simulink model "ComplexLS"  (R2018b)
settings: Solver=FixedStepAuto  StartTime=1  StopTime=10  FixedStep=1  RelTol=1e-3
libraries: hdlsllib x11, simulink x1
settings Model: Creator=jason  LastModifiedBy=jason
settings OptimizationCC: DefaultParameterBehavior=Inlined

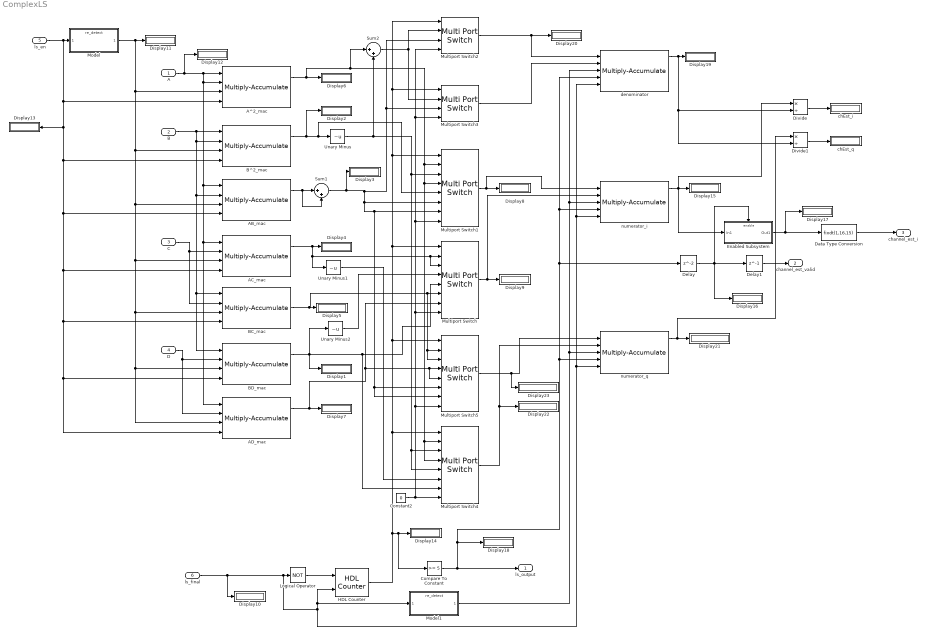
== system ComplexLS ==
  A : Inport  OutDataTypeStr=fixdt(1,16,15)  SampleTime=1  Interpolate=off
  B : Inport  Port=2  OutDataTypeStr=fixdt(1,16,15)  SampleTime=1  Interpolate=off
  C : Inport  Port=3  OutDataTypeStr=fixdt(1,16,15)  SampleTime=1  Interpolate=off
  D : Inport  Port=4  OutDataTypeStr=fixdt(1,16,15)  SampleTime=1  Interpolate=off
  ls_en : Inport  Port=5  OutDataTypeStr=boolean
  ls_final : Inport  Port=6  OutDataTypeStr=boolean
  AB_mac : hdlsllib/HDL Operations/Multiply-Accumulate  opMode=Streaming - using Start and End ports  initValueSetting=Dialog  initValue=0  initValueSetting2=Dialog  initValue2=0  initValueSetting3=Dialog  initValue3=0  num_samples=2  RndMeth2=Floor  RndMeth3=Floor  datatype2=fixdt(1,64,32)  datatype3=Inherit: Inherit via back propagation  validOut=on  endInandOut=off  startOut=off  countOut=on  dim=-1  DoSatur=off  parallel=off
      settings: SourceProductName=HDL Coder  SourceProductBaseCode=HD
  AC_mac : hdlsllib/HDL Operations/Multiply-Accumulate  opMode=Streaming - using Start and End ports  initValueSetting=Dialog  initValue=0  initValueSetting2=Dialog  initValue2=0  initValueSetting3=Dialog  initValue3=0  num_samples=2  RndMeth2=Floor  RndMeth3=Floor  datatype2=fixdt(1,64,32)  datatype3=Inherit: Inherit via back propagation  validOut=on  endInandOut=off  startOut=off  countOut=on  dim=-1  DoSatur=off  parallel=off
      settings: SourceProductName=HDL Coder  SourceProductBaseCode=HD
  AD_mac : hdlsllib/HDL Operations/Multiply-Accumulate  opMode=Streaming - using Start and End ports  initValueSetting=Dialog  initValue=0  initValueSetting2=Dialog  initValue2=0  initValueSetting3=Dialog  initValue3=0  num_samples=2  RndMeth2=Floor  RndMeth3=Floor  datatype2=fixdt(1,64,32)  datatype3=Inherit: Inherit via back propagation  validOut=on  endInandOut=off  startOut=off  countOut=on  dim=-1  DoSatur=off  parallel=off
      settings: SourceProductName=HDL Coder  SourceProductBaseCode=HD
  A^2_mac : hdlsllib/HDL Operations/Multiply-Accumulate  opMode=Streaming - using Start and End ports  initValueSetting=Dialog  initValue=0  initValueSetting2=Dialog  initValue2=0  initValueSetting3=Dialog  initValue3=0  num_samples=2  RndMeth2=Floor  RndMeth3=Floor  datatype2=fixdt(1,64,32)  datatype3=Inherit: Inherit via back propagation  validOut=on  endInandOut=off  startOut=off  countOut=on  dim=-1  DoSatur=off  parallel=off
      settings: SourceProductName=HDL Coder  SourceProductBaseCode=HD
  BC_mac : hdlsllib/HDL Operations/Multiply-Accumulate  opMode=Streaming - using Start and End ports  initValueSetting=Dialog  initValue=0  initValueSetting2=Dialog  initValue2=0  initValueSetting3=Dialog  initValue3=0  num_samples=2  RndMeth2=Floor  RndMeth3=Floor  datatype2=fixdt(1,64,32)  datatype3=Inherit: Inherit via back propagation  validOut=off  endInandOut=off  startOut=off  countOut=on  dim=-1  DoSatur=off  parallel=off
      settings: SourceProductName=HDL Coder  SourceProductBaseCode=HD
  BD_mac : hdlsllib/HDL Operations/Multiply-Accumulate  opMode=Streaming - using Start and End ports  initValueSetting=Dialog  initValue=0  initValueSetting2=Dialog  initValue2=0  initValueSetting3=Dialog  initValue3=0  num_samples=2  RndMeth2=Floor  RndMeth3=Floor  datatype2=fixdt(1,64,32)  datatype3=Inherit: Inherit via back propagation  validOut=on  endInandOut=off  startOut=off  countOut=on  dim=-1  DoSatur=off  parallel=off
      settings: SourceProductName=HDL Coder  SourceProductBaseCode=HD
  B^2_mac : hdlsllib/HDL Operations/Multiply-Accumulate  opMode=Streaming - using Start and End ports  initValueSetting=Dialog  initValue=0  initValueSetting2=Dialog  initValue2=0  initValueSetting3=Dialog  initValue3=0  num_samples=2  RndMeth2=Floor  RndMeth3=Floor  datatype2=fixdt(1,64,32)  datatype3=Inherit: Inherit via back propagation  validOut=on  endInandOut=off  startOut=off  countOut=on  dim=-1  DoSatur=off  parallel=off
      settings: SourceProductName=HDL Coder  SourceProductBaseCode=HD
  Compare To Constant : simulink/Logic and Bit Operations/Compare To Constant  relop=>=  const=5  OutDataTypeStr=boolean
  Constant2 : Constant  Value=0  OutDataTypeStr=fixdt(1,64,32)  SampleTime=-1
  Data Type Conversion : DataTypeConversion  OutDataTypeStr=fixdt(1,16,15)
  Delay : Delay
  Delay1 : Delay  DelayLength=1
  Display{1..23} (23 alike) : Display
  Divide : Product  Inputs=*/  OutDataTypeStr=double  SaturateOnIntegerOverflow=on  RndMeth=Zero
  Divide1 : Product  Inputs=*/  OutDataTypeStr=double  SaturateOnIntegerOverflow=on  RndMeth=Zero
  Enabled Subsystem : Subsystem  TreatAsAtomicUnit=on
  HDL Counter : hdlsllib/Sources/HDL Counter  CountType=Count limited  CountInit=0  CountStep=1  CountMax=5  CountFromType=Initial value  CountFrom=0  CountResetPort=on  CountLoadPort=off  CountEnbPort=on  CountDirPort=off  CountDataType=Unsigned  CountWordLen=8  CountFracLen=0  CountSampTime=1
      settings: SourceProductBaseCode=HD
  Logical Operator : Logic  Operator=NOT  IconShape=distinctive  AllPortsSameDT=off  OutDataTypeStr=boolean
  Model : ModelReference  ModelNameDialog=re_detect.slx  SimulationMode=Normal  ModelReferenceVersion=1.5
  Model1 : ModelReference  ModelNameDialog=re_detect.slx  SimulationMode=Normal  ModelReferenceVersion=1.5
  Multiport Switch : MultiPortSwitch  DataPortOrder=Zero-based contiguous  Inputs=6  DataPortIndices={0,1,2,3,4,5}  DataPortForDefault=Additional data port  zeroidx=on  InputSameDT=on
  Multiport Switch1 : MultiPortSwitch  DataPortOrder=Zero-based contiguous  Inputs=6  DataPortIndices=uint8({0,1,2,3,4,5})  DataPortForDefault=Additional data port  zeroidx=on  InputSameDT=on
  Multiport Switch2 : MultiPortSwitch  DataPortOrder=Zero-based contiguous  Inputs=2  DataPortIndices=uint8({0,1,2,3,4,5})  DataPortForDefault=Additional data port  DiagnosticForDefault=None  zeroidx=on  InputSameDT=on
  Multiport Switch3 : MultiPortSwitch  DataPortOrder=Zero-based contiguous  Inputs=2  DataPortIndices=uint8({0,1,2,3,4,5})  DataPortForDefault=Additional data port  DiagnosticForDefault=None  zeroidx=on  InputSameDT=on
  Multiport Switch4 : MultiPortSwitch  DataPortOrder=Zero-based contiguous  Inputs=6  DataPortIndices={0,1,2,3,4,5}  DataPortForDefault=Additional data port  zeroidx=on  InputSameDT=on
  Multiport Switch5 : MultiPortSwitch  DataPortOrder=Zero-based contiguous  Inputs=6  DataPortIndices=uint8({0,1,2,3,4,5})  DataPortForDefault=Additional data port  zeroidx=on  InputSameDT=on
  Sum1 : Sum  Inputs=|++
  Sum2 : Sum  Inputs=|++
  Unary Minus : UnaryMinus
  Unary Minus1 : UnaryMinus
  Unary Minus2 : UnaryMinus
  chEst_i : Display
  chEst_q : Display
  denominator : hdlsllib/HDL Operations/Multiply-Accumulate  opMode=Streaming - using Start and End ports  initValueSetting=Dialog  initValue=0  initValueSetting2=Dialog  initValue2=0  initValueSetting3=Dialog  initValue3=0  num_samples=2  RndMeth2=Floor  RndMeth3=Floor  datatype2=Inherit: Inherit via back propagation  datatype3=Inherit: Inherit via back propagation  validOut=on  endInandOut=on  startOut=off  countOut=on  dim=-1  DoSatur=off  parallel=off
      settings: SourceProductName=HDL Coder  SourceProductBaseCode=HD
  numerator_i : hdlsllib/HDL Operations/Multiply-Accumulate  opMode=Streaming - using Start and End ports  initValueSetting=Dialog  initValue=0  initValueSetting2=Dialog  initValue2=0  initValueSetting3=Dialog  initValue3=0  num_samples=2  RndMeth2=Floor  RndMeth3=Floor  datatype2=Inherit: Inherit via back propagation  datatype3=Inherit: Inherit via back propagation  validOut=on  endInandOut=on  startOut=off  countOut=on  dim=-1  DoSatur=off  parallel=off
      settings: SourceProductName=HDL Coder  SourceProductBaseCode=HD
  numerator_q : hdlsllib/HDL Operations/Multiply-Accumulate  opMode=Streaming - using Start and End ports  initValueSetting=Dialog  initValue=0  initValueSetting2=Dialog  initValue2=0  initValueSetting3=Dialog  initValue3=0  num_samples=2  RndMeth2=Floor  RndMeth3=Floor  datatype2=Inherit: Inherit via back propagation  datatype3=Inherit: Inherit via back propagation  validOut=on  endInandOut=on  startOut=off  countOut=on  dim=-1  DoSatur=off  parallel=off
      settings: SourceProductName=HDL Coder  SourceProductBaseCode=HD
  ls_output : Outport  OutDataTypeStr=boolean
  channel_est_valid : Outport  Port=2  OutDataTypeStr=boolean
  channel_est_i : Outport  Port=3  OutDataTypeStr=fixdt(1,16,15)
  wires:
  A/1 -> Display12/1, A^2_mac/1, AB_mac/1, AC_mac/1, AD_mac/1, A^2_mac/2
  B/1 -> B^2_mac/1, BD_mac/1, BC_mac/1, AB_mac/2, B^2_mac/2
  C/1 -> BC_mac/2, AC_mac/2
  D/1 -> AD_mac/2, BD_mac/2
  ls_en/1 -> Display13/1, AD_mac/4, BD_mac/4, BC_mac/4, AC_mac/4, AB_mac/4, B^2_mac/4, A^2_mac/4, Model/1
  Model/1 -> Display11/1, AD_mac/3, BD_mac/3, BC_mac/3, AC_mac/3, AB_mac/3, B^2_mac/3, A^2_mac/3
  AD_mac/1 -> Multiport Switch5/5, Multiport Switch5/4, Multiport Switch/7, Display7/1
  BD_mac/1 -> Unary Minus2/1, Multiport Switch/5, Multiport Switch4/7, Display1/1
  BC_mac/1 -> Multiport Switch5/2, Multiport Switch5/3, Multiport Switch/6, Display5/1
  AC_mac/1 -> Unary Minus1/1, Multiport Switch/2, Multiport Switch/3, Display4/1
  AB_mac/1 -> Sum1/2, Sum1/1
  B^2_mac/1 -> Display2/1, Multiport Switch1/5, Unary Minus/1
  A^2_mac/1 -> Display6/1, Multiport Switch4/2, Multiport Switch4/4, Multiport Switch1/4, Multiport Switch1/2, Sum2/1
  Constant2/1 -> Multiport Switch4/8, Multiport Switch5/8, Multiport Switch/8, Multiport Switch1/8, Multiport Switch3/4, Multiport Switch2/4
  Unary Minus/1 -> Multiport Switch4/3, Multiport Switch4/5, Multiport Switch1/3, Sum2/2
  Multiport Switch/1 -> numerator_i/2, Display9/1
  Multiport Switch1/1 -> numerator_i/1, Display8/1
  ls_final/1 -> HDL Counter/2, Model1/1, denominator/5, numerator_i/5, numerator_q/5, Logical Operator/1, Display10/1
  Logical Operator/1 -> HDL Counter/1
  HDL Counter/1 -> Compare To Constant/1, Display14/1, Multiport Switch4/1, Multiport Switch5/1, Multiport Switch/1, Multiport Switch3/1, Multiport Switch2/1, Multiport Switch1/1
  numerator_i/1 -> Divide/1, Enabled Subsystem/1(In1), Display15/1
  Compare To Constant/1 -> ls_output/1, Display18/1, denominator/4, numerator_i/4, Delay/1, numerator_q/4
  Delay/1 -> Delay1/1, Enabled Subsystem/Enable, Display16/1
  Enabled Subsystem/1(Out1) -> Data Type Conversion/1, Display17/1
  Delay1/1 -> channel_est_valid/1
  Sum1/1 -> Multiport Switch1/7, Multiport Switch5/7, Multiport Switch5/6, Multiport Switch1/6, Multiport Switch3/3, Multiport Switch2/3, Display3/1
  Sum2/1 -> Multiport Switch2/2, Multiport Switch3/2
  Multiport Switch2/1 -> Display20/1, denominator/1
  Multiport Switch3/1 -> denominator/2
  denominator/1 -> Divide1/2, Divide/2, Display19/1
  Multiport Switch5/1 -> Display23/1, numerator_q/1
  Multiport Switch4/1 -> Display22/1, numerator_q/2
  numerator_q/1 -> Divide1/1, Display21/1
  Unary Minus2/1 -> Multiport Switch/4
  Divide/1 -> chEst_i/1
  Divide1/1 -> chEst_q/1
  Model1/1 -> denominator/3, numerator_i/3, numerator_q/3
  Unary Minus1/1 -> Multiport Switch4/6
  Data Type Conversion/1 -> channel_est_i/1

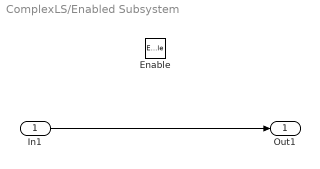
== system ComplexLS/Enabled Subsystem ==
  In1 : Inport
  Enable : EnablePort
  Out1 : Outport  InitialOutput=0
  wires:
  In1/1 -> Out1/1
